simulink model "Battery_Management_System"  (R2025a)
settings: Solver=VariableStepAuto  StartTime=0.0  StopTime=50  RelTol=1e-3
libraries: SignalEditorBlockLib x1
settings Model: Creator=Rudransh  LastModifiedBy=Rudransh

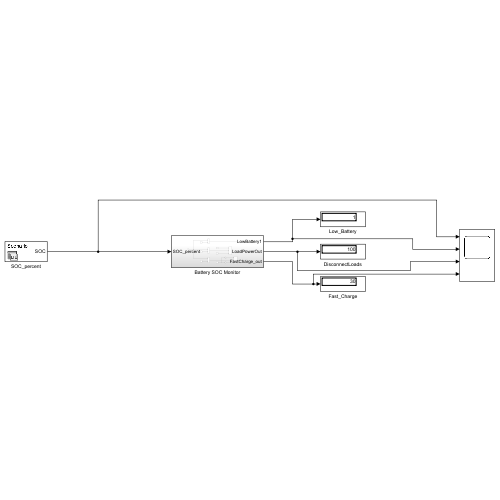
[thumbnail: Simulink's stored preview of the top-level diagram]
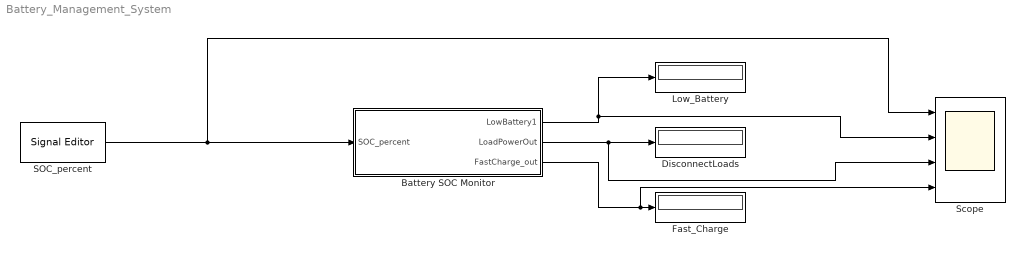
== system Battery_Management_System ==
  Battery SOC Monitor : Subsystem
  DisconnectLoads : Display
  Fast_Charge : Display
  Low_Battery : Display
  SOC_percent : SignalEditorBlockLib/Signal Editor  FileName=C:\Projects_ESD\AUTOSAR_CARSYSTEM\Battery_Management\Scenario\Scenario2.mat  ActiveScenario=Scenario  ActiveSignal=SOC  IsBus=off  OutputBusObjectStr=Bus: BusObject  SampleTime=0  ZeroCross=off  OutputAfterFinalValue=Setting to zero  Unit=inherit  PreserveSignalName=on  ApplySigPropsToAllScenarios=on  ApplySigPropsToAllSignals=off  SignalPropertySource=Dialog parameters
  Scope : Scope  NumInputPorts=4
      settings: ActiveDisplayString=4  Title=BatterySOCMonitor3  ActiveDisplayYMinimum=7.5000000000000009  ActiveDisplayYMaximum=32.5
  wires:
  Battery SOC Monitor/1(LowBattery1) -> Low_Battery/1, Scope/2
  Battery SOC Monitor/2(LoadPowerOut) -> Scope/3, DisconnectLoads/1
  Battery SOC Monitor/3(FastCharge_out) -> Scope/4, Fast_Charge/1
  SOC_percent/1 -> Scope/1, Battery SOC Monitor/1(SOC_percent)

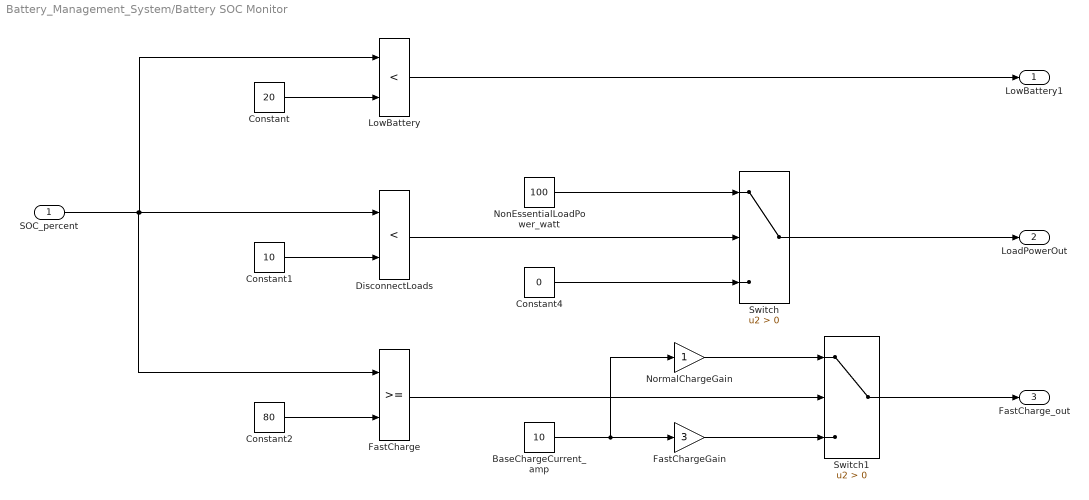
== system Battery_Management_System/Battery SOC Monitor ==
  SOC_percent : Inport
  BaseChargeCurrent_amp : Constant  Value=10
  Constant : Constant  Value=20
  Constant1 : Constant  Value=10
  Constant2 : Constant  Value=80
  Constant4 : Constant  Value=0
  DisconnectLoads : RelationalOperator  Operator=<  OutDataTypeStr=boolean  RndMeth=Simplest  InputSameDT=off
  FastCharge : RelationalOperator  OutDataTypeStr=boolean  RndMeth=Simplest  InputSameDT=off
  FastChargeGain : Gain  Gain=3
  LowBattery : RelationalOperator  Operator=<  OutDataTypeStr=boolean  RndMeth=Simplest  InputSameDT=off
  NonEssentialLoadPower_watt : Constant  Value=100
  NormalChargeGain : Gain
  Switch : Switch  Criteria=u2 > Threshold  SaturateOnIntegerOverflow=off  InputSameDT=off
  Switch1 : Switch  Criteria=u2 > Threshold  SaturateOnIntegerOverflow=off  InputSameDT=off
  LowBattery1 : Outport
  LoadPowerOut : Outport  Port=2
  FastCharge_out : Outport  Port=3
  wires:
  BaseChargeCurrent_amp/1 -> NormalChargeGain/1, FastChargeGain/1
  SOC_percent/1 -> FastCharge/1, LowBattery/1, DisconnectLoads/1
  NormalChargeGain/1 -> Switch1/1
  Constant2/1 -> FastCharge/2
  Constant1/1 -> DisconnectLoads/2
  FastChargeGain/1 -> Switch1/3
  Switch1/1 -> FastCharge_out/1
  Constant/1 -> LowBattery/2
  NonEssentialLoadPower_watt/1 -> Switch/1
  Constant4/1 -> Switch/3
  DisconnectLoads/1 -> Switch/2
  LowBattery/1 -> LowBattery1/1
  FastCharge/1 -> Switch1/2
  Switch/1 -> LoadPowerOut/1
